simulink model "SimpleSubSystem"  (Simulink 7.4)
settings: Solver=ode45  StartTime=0.0  StopTime=10.0  RelTol=1e-3
settings Model: Creator=dread  LastModifiedBy=dread

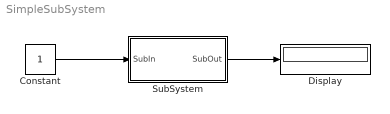
== system SimpleSubSystem ==
  Constant : Constant  OutDataType=fixdt(1, 16)  OutScaling=2^0
  Display : Display
  SubSystem : Subsystem  Tag=id=_SUBSYSTEMTESTIDgVdmhug
  wires:
  Constant/1 -> SubSystem/1(SubIn)
  SubSystem/1(SubOut) -> Display/1

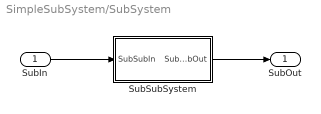
== system SimpleSubSystem/SubSystem ==
  SubIn : Inport  OutDataType=fixdt(1, 16)  OutScaling=2^0
  SubSubSystem : Subsystem  Tag=id=_SUBSUBSYSTEMTESTIDgVdm
  SubOut : Outport  OutDataType=fixdt(1, 16)  OutScaling=2^0
  wires:
  SubIn/1 -> SubSubSystem/1(SubSubIn)
  SubSubSystem/1(SubSubOut) -> SubOut/1

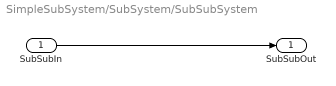
== system SimpleSubSystem/SubSystem/SubSubSystem ==
  SubSubIn : Inport  OutDataType=fixdt(1, 16)  OutScaling=2^0
  SubSubOut : Outport  OutDataType=fixdt(1, 16)  OutScaling=2^0
  wires:
  SubSubIn/1 -> SubSubOut/1
